simulink model "pmsm_current_loop_discrete"  (R2024b)
settings: Solver=FixedStepDiscrete  StartTime=0.0  StopTime=0.05  FixedStep=Ts  RelTol=1e-3
InitFcn:
  | model_file = get_param(bdroot, 'FileName');
  | model_dir = fileparts(model_file);
  | run(fullfile(model_dir, 'pmsm_current_loop_params.m'));
values from neighbouring files (symbols this model uses):
  flux_wb = 0.0078    [pmsm_current_loop_params.m]
  id_ki = iq_ki * 0.2    (= 666)    [pmsm_current_loop_params.m]
  id_kp = iq_kp * 0.5    (= 1.885)    [pmsm_current_loop_params.m]
  id_ref_after = id_ref_a_default    (= 0)    [pmsm_current_loop_params.m]
  id_ref_before = 0.0    (= 0)    [pmsm_current_loop_params.m]
  id_ref_step_time = 0.001    [pmsm_current_loop_params.m]
  iq_ki = 3330.0    (= 3330)    [pmsm_current_loop_params.m]
  iq_kp = 3.770    (= 3.77)    [pmsm_current_loop_params.m]
  iq_ref_after = iq_ref_a_default    (= 1)    [pmsm_current_loop_params.m]
  iq_ref_before = 0.0    (= 0)    [pmsm_current_loop_params.m]
  iq_ref_step_time = 0.001    [pmsm_current_loop_params.m]
  Ld = 0.0006    [pmsm_current_loop_params.m]
  Lq = 0.0006    [pmsm_current_loop_params.m]
  plant_vd_effect_sign = -1.0    (= -1)    [pmsm_current_loop_params.m]
  plant_vq_effect_sign = -1.0    (= -1)    [pmsm_current_loop_params.m]
  pole_pairs = 4.0    (= 4)    [pmsm_current_loop_params.m]
  pwm_arr = 5311.0    (= 5311)    [pmsm_current_loop_params.m]
  Rs = 0.53    [pmsm_current_loop_params.m]
  sim_mech_speed_rad_s = 50.0    (= 50)    [pmsm_current_loop_params.m]
  svpwm_max_ccr = pwm_arr - 20.0    (= 5291)    [pmsm_current_loop_params.m]
  svpwm_min_ccr = 20.0    (= 20)    [pmsm_current_loop_params.m]
  Ts = 6.25e-5    (= 6.25e-05)    [pmsm_current_loop_params.m]
  use_svpwm_equivalent = 0    [pmsm_current_loop_params.m]
  v_limit = 13.5    [pmsm_current_loop_params.m]
  Vbus = 24.0    (= 24)    [pmsm_current_loop_params.m]
  vd_cmd_sign = -1.0    (= -1)    [pmsm_current_loop_params.m]
  vq_cmd_sign = -1.0    (= -1)    [pmsm_current_loop_params.m]
Description:
  | PMSM discrete current-loop verification model.
  | Parameters are loaded from model/simulink/pmsm_current_loop_params.m.
  | use_svpwm_equivalent=0 bypasses SVPWM and feeds InvPark voltage directly to the plant.
  | use_svpwm_equivalent=1 uses the C-like SVPWM/inverter equivalent before the plant.
  | No observer, PLL, handover, startup, speed loop, or Simscape power bridge is included.
settings Model: Creator=10095  LastModifiedBy=10095
settings DataIOCC: SaveFormat=StructureWithTime

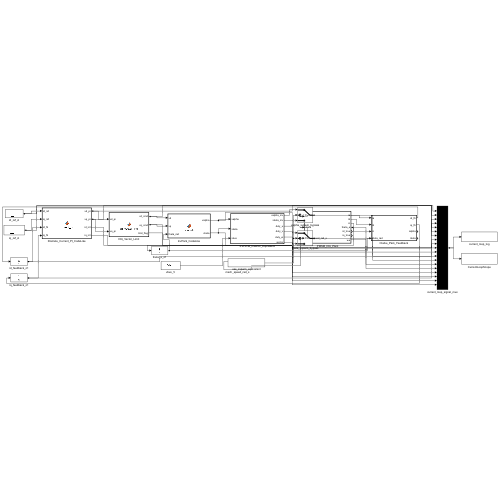
[thumbnail: Simulink's stored preview of the top-level diagram]
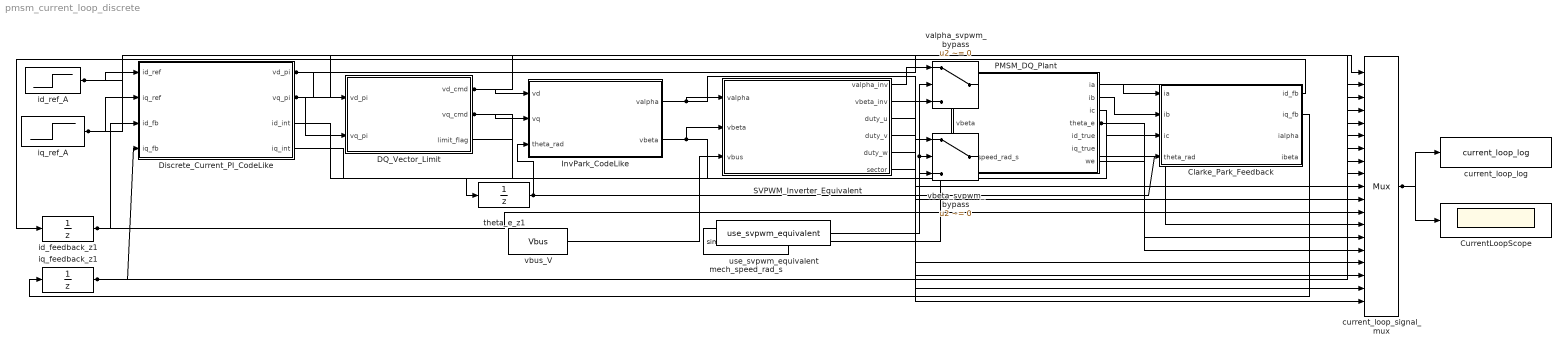
== system pmsm_current_loop_discrete ==
  Clarke_Park_Feedback : MATLAB Function  TreatAsAtomicUnit=on
  CurrentLoopScope : Scope
  DQ_Vector_Limit : MATLAB Function  TreatAsAtomicUnit=on
  Discrete_Current_PI_CodeLike : MATLAB Function  TreatAsAtomicUnit=on
  InvPark_CodeLike : MATLAB Function  TreatAsAtomicUnit=on
  PMSM_DQ_Plant : MATLAB Function  TreatAsAtomicUnit=on
  SVPWM_Inverter_Equivalent : MATLAB Function  TreatAsAtomicUnit=on
  current_loop_log : ToWorkspace  VariableName=current_loop_log  SampleTime=-1
  current_loop_signal_mux : Mux  Inputs=19
  id_feedback_z1 : UnitDelay  SampleTime=Ts  HasFrameUpgradeWarning=on
  id_ref_A : Step  Time=id_ref_step_time  Before=id_ref_before  After=id_ref_after  SampleTime=Ts
  iq_feedback_z1 : UnitDelay  SampleTime=Ts  HasFrameUpgradeWarning=on
  iq_ref_A : Step  Time=iq_ref_step_time  Before=iq_ref_before  After=iq_ref_after  SampleTime=Ts
  mech_speed_rad_s : Constant  Value=sim_mech_speed_rad_s
  theta_e_z1 : UnitDelay  SampleTime=Ts  HasFrameUpgradeWarning=on
  use_svpwm_equivalent : Constant  Value=use_svpwm_equivalent
  valpha_svpwm_bypass : Switch  Criteria=u2 ~= 0  Threshold=0.5  SaturateOnIntegerOverflow=off  InputSameDT=off
  vbeta_svpwm_bypass : Switch  Criteria=u2 ~= 0  Threshold=0.5  SaturateOnIntegerOverflow=off  InputSameDT=off
  vbus_V : Constant  Value=Vbus
  wires:
  id_ref_A/1 -> Discrete_Current_PI_CodeLike/1(id_ref), current_loop_signal_mux/1
  iq_ref_A/1 -> Discrete_Current_PI_CodeLike/2(iq_ref), current_loop_signal_mux/2
  id_feedback_z1/1 -> Discrete_Current_PI_CodeLike/3(id_fb), current_loop_signal_mux/3
  iq_feedback_z1/1 -> Discrete_Current_PI_CodeLike/4(iq_fb), current_loop_signal_mux/4
  Discrete_Current_PI_CodeLike/1(vd_pi) -> DQ_Vector_Limit/1(vd_pi), current_loop_signal_mux/5
  Discrete_Current_PI_CodeLike/2(vq_pi) -> DQ_Vector_Limit/2(vq_pi), current_loop_signal_mux/6
  DQ_Vector_Limit/1(vd_cmd) -> InvPark_CodeLike/1(vd), current_loop_signal_mux/7
  DQ_Vector_Limit/2(vq_cmd) -> InvPark_CodeLike/2(vq), current_loop_signal_mux/8
  theta_e_z1/1 -> InvPark_CodeLike/3(theta_rad), Clarke_Park_Feedback/4(theta_rad)
  InvPark_CodeLike/1(valpha) -> SVPWM_Inverter_Equivalent/1(valpha), valpha_svpwm_bypass/3
  InvPark_CodeLike/2(vbeta) -> SVPWM_Inverter_Equivalent/2(vbeta), vbeta_svpwm_bypass/3
  vbus_V/1 -> SVPWM_Inverter_Equivalent/3(vbus)
  mech_speed_rad_s/1 -> PMSM_DQ_Plant/3(mech_speed_rad_s)
  PMSM_DQ_Plant/1(ia) -> Clarke_Park_Feedback/1(ia)
  PMSM_DQ_Plant/2(ib) -> Clarke_Park_Feedback/2(ib)
  PMSM_DQ_Plant/3(ic) -> Clarke_Park_Feedback/3(ic)
  Clarke_Park_Feedback/1(id_fb) -> id_feedback_z1/1
  Clarke_Park_Feedback/2(iq_fb) -> iq_feedback_z1/1
  PMSM_DQ_Plant/4(theta_e) -> theta_e_z1/1, current_loop_signal_mux/14
  SVPWM_Inverter_Equivalent/1(valpha_inv) -> valpha_svpwm_bypass/1
  use_svpwm_equivalent/1 -> valpha_svpwm_bypass/2, vbeta_svpwm_bypass/2
  SVPWM_Inverter_Equivalent/2(vbeta_inv) -> vbeta_svpwm_bypass/1
  valpha_svpwm_bypass/1 -> PMSM_DQ_Plant/1(valpha), current_loop_signal_mux/12
  vbeta_svpwm_bypass/1 -> PMSM_DQ_Plant/2(vbeta), current_loop_signal_mux/13
  DQ_Vector_Limit/3(limit_flag) -> current_loop_signal_mux/9
  Discrete_Current_PI_CodeLike/3(id_int) -> current_loop_signal_mux/10
  Discrete_Current_PI_CodeLike/4(iq_int) -> current_loop_signal_mux/11
  PMSM_DQ_Plant/7(we) -> current_loop_signal_mux/15
  SVPWM_Inverter_Equivalent/3(duty_u) -> current_loop_signal_mux/16
  SVPWM_Inverter_Equivalent/4(duty_v) -> current_loop_signal_mux/17
  SVPWM_Inverter_Equivalent/5(duty_w) -> current_loop_signal_mux/18
  SVPWM_Inverter_Equivalent/6(sector) -> current_loop_signal_mux/19
  current_loop_signal_mux/1 -> current_loop_log/1, CurrentLoopScope/1

== matlab function pmsm_current_loop_discrete/PMSM_DQ_Plant ==
  data: valpha input; ia output; vbeta input; mech_speed_rad_s input; ib output; ic output; theta_e output; id_true output; iq_true output; we output; pole_pairs parameter; Ts parameter; Rs parameter; Ld parameter; Lq parameter; flux_wb parameter; plant_vd_effect_sign parameter; plant_vq_effect_sign parameter
function [ia, ib, ic, theta_e, id_true, iq_true, we] = pmsm_plant(valpha, vbeta, mech_speed_rad_s, pole_pairs, Ts, Rs, Ld, Lq, flux_wb, plant_vd_effect_sign, plant_vq_effect_sign)
%#codegen
persistent id_state iq_state theta
ia = 0.0; ib = 0.0; ic = 0.0;
theta_e = 0.0; id_true = 0.0; iq_true = 0.0; we = 0.0;
if isempty(id_state)
    id_state = 0.0;
    iq_state = 0.0;
    theta = 0.0;
end
we = pole_pairs * mech_speed_rad_s;
theta_e = theta;
s = sin(theta_e);
c = cos(theta_e);
% C reference: ClarkePark_Park() in foc_clarke_park.c.
vd_cmd = (valpha * c) + (vbeta * s);
vq_cmd = (-valpha * s) + (vbeta * c);
% Plant-side polarity adapter only. The control-side negative signs are
% vd_cmd_sign/vq_cmd_sign in foc_current_loop.c, not hidden here.
vd = plant_vd_effect_sign * vd_cmd;
vq = plant_vq_effect_sign * vq_cmd;
did = (vd - (Rs * id_state) + (we * Lq * iq_state)) / Ld;
diq = (vq - (Rs * iq_state) - (we * Ld * id_state) - (we * flux_wb)) / Lq;
id_state = id_state + (Ts * did);
iq_state = iq_state + (Ts * diq);
theta = theta + (we * Ts);
theta = theta - (floor(theta / 6.283185307179586) * 6.283185307179586);
id_true = id_state;
iq_true = iq_state;
ialpha = (id_state * c) - (iq_state * s);
ibeta = (id_state * s) + (iq_state * c);
ia = ialpha;
ib = (-0.5 * ialpha) + (0.8660254 * ibeta);
ic = (-0.5 * ialpha) - (0.8660254 * ibeta);
end

== matlab function pmsm_current_loop_discrete/Clarke_Park_Feedback ==
  data: ia input; id_fb output; ib input; ic input; theta_rad input; iq_fb output; ialpha output; ibeta output
function [id_fb, iq_fb, ialpha, ibeta] = clarke_park_feedback(ia, ib, ic, theta_rad)
%#codegen
id_fb = 0.0; iq_fb = 0.0; ialpha = 0.0; ibeta = 0.0;
unused_ic = ic;
% C reference: ClarkePark_Clarke() in foc_clarke_park.c.
ialpha = ia;
ibeta = (ia + (2.0 * ib)) * 0.577350269;
s = sin(theta_rad);
c = cos(theta_rad);
% C reference: ClarkePark_Park() in foc_clarke_park.c.
id_fb = (ialpha * c) + (ibeta * s);
iq_fb = (-ialpha * s) + (ibeta * c);
if unused_ic ~= unused_ic
    id_fb = id_fb;
end
end

== matlab function pmsm_current_loop_discrete/DQ_Vector_Limit ==
  data: vd_pi input; vd_cmd output; vq_pi input; vq_cmd output; limit_flag output; dq_v_limit parameter
function [vd_cmd, vq_cmd, limit_flag] = dq_vector_limit(vd_pi, vq_pi, dq_v_limit)
%#codegen
vd_cmd = 0.0; vq_cmd = 0.0; limit_flag = 0.0;
mag_sq = (vd_pi * vd_pi) + (vq_pi * vq_pi);
limit_sq = dq_v_limit * dq_v_limit;
if mag_sq > limit_sq
    scale = dq_v_limit / sqrt(mag_sq);
    vd_cmd = vd_pi * scale;
    vq_cmd = vq_pi * scale;
    limit_flag = 1.0;
else
    vd_cmd = vd_pi;
    vq_cmd = vq_pi;
    limit_flag = 0.0;
end
end

== matlab function pmsm_current_loop_discrete/Discrete_Current_PI_CodeLike ==
  data: id_ref input; vd_pi output; iq_ref input; id_fb input; iq_fb input; vq_pi output; id_int output; iq_int output; id_kp parameter; id_ki parameter; iq_kp parameter; iq_ki parameter; Ts parameter; v_limit parameter; vd_cmd_sign parameter; vq_cmd_sign parameter
function [vd_pi, vq_pi, id_int, iq_int] = current_pi(id_ref, iq_ref, id_fb, iq_fb, id_kp, id_ki, iq_kp, iq_ki, Ts, v_limit, vd_cmd_sign, vq_cmd_sign)
%#codegen
persistent id_integral iq_integral
vd_pi = 0.0; vq_pi = 0.0; id_int = 0.0; iq_int = 0.0;
if isempty(id_integral)
    id_integral = 0.0;
    iq_integral = 0.0;
end
[id_out, id_integral] = pi_run(id_ref, id_fb, id_kp, id_ki, id_integral, Ts, v_limit);
[iq_out, iq_integral] = pi_run(iq_ref, iq_fb, iq_kp, iq_ki, iq_integral, Ts, v_limit);
% C reference: foc_current_loop.c multiplies PI output by FOC_VD_CMD_SIGN.
vd_pi = vd_cmd_sign * id_out;
% C reference: foc_current_loop.c multiplies PI output by FOC_VQ_CMD_SIGN.
vq_pi = vq_cmd_sign * iq_out;
id_int = id_integral;
iq_int = iq_integral;
end

function [out, integral] = pi_run(ref, meas, kp, ki, integral, dt_sec, limit)
err = ref - meas;
p_term = kp * err;
integral_next = integral + (ki * err * dt_sec);
integral_next = clampf(integral_next, -limit, limit);
unsat = p_term + integral_next;
out = clampf(unsat, -limit, limit);
if ((unsat == out) || ((unsat > limit) && (err < 0.0)) || ((unsat < -limit) && (err > 0.0)))
    integral = integral_next;
end
end

function y = clampf(x, mn, mx)
if x > mx
    y = mx;
elseif x < mn
    y = mn;
else
    y = x;
end
end

== matlab function pmsm_current_loop_discrete/InvPark_CodeLike ==
  data: vd input; valpha output; vq input; theta_rad input; vbeta output
function [valpha, vbeta] = invpark(vd, vq, theta_rad)
%#codegen
valpha = 0.0; vbeta = 0.0;
s = sin(theta_rad);
c = cos(theta_rad);
% C reference: ClarkePark_InvPark() in foc_clarke_park.c.
valpha = (vd * c) - (vq * s);
vbeta = (vd * s) + (vq * c);
end

== matlab function pmsm_current_loop_discrete/SVPWM_Inverter_Equivalent ==
  data: valpha input; valpha_inv output; vbeta input; vbus input; vbeta_inv output; duty_u output; duty_v output; duty_w output; sector output; pwm_arr parameter; Vbus parameter; svpwm_min_ccr parameter; svpwm_max_ccr parameter
function [valpha_inv, vbeta_inv, duty_u, duty_v, duty_w, sector] = svpwm_inverter(valpha, vbeta, vbus, pwm_arr, Vbus, svpwm_min_ccr, svpwm_max_ccr)
%#codegen
valpha_inv = 0.0; vbeta_inv = 0.0;
duty_u = 0.5; duty_v = 0.5; duty_w = 0.5; sector = 1.0;
two_pi = 6.283185307179586;
pi_over_3 = 1.047197551196598;
sqrt3 = 1.732050807568877;
pwm_period = pwm_arr;
angle = atan2(vbeta, valpha);
if angle < 0.0
    angle = angle + two_pi;
end
sector = floor(angle * 0.95492965855) + 1.0;
if sector > 6.0
    sector = 6.0;
end
norm_vbus = vbus;
if norm_vbus <= 0.1
    norm_vbus = Vbus;
end
theta_sector = angle - ((sector - 1.0) * pi_over_3);
if theta_sector < 0.0
    theta_sector = 0.0;
elseif theta_sector > pi_over_3
    theta_sector = pi_over_3;
end
vref = sqrt((valpha * valpha) + (vbeta * vbeta));
t1 = pwm_period * sqrt3 * (vref / norm_vbus) * sin(pi_over_3 - theta_sector);
t2 = pwm_period * sqrt3 * (vref / norm_vbus) * sin(theta_sector);
if t1 < 0.0, t1 = 0.0; end
if t2 < 0.0, t2 = 0.0; end
if (t1 + t2) > pwm_period
    scale = pwm_period / (t1 + t2);
    t1 = t1 * scale;
    t2 = t2 * scale;
end
t0 = pwm_period - t1 - t2;
if t0 < 0.0, t0 = 0.0; end
half_t0 = 0.5 * t0;
if sector == 1.0
    ta = t1 + t2 + half_t0; tb = t2 + half_t0;      tc = half_t0;
elseif sector == 2.0
    ta = t1 + half_t0;      tb = t1 + t2 + half_t0; tc = half_t0;
elseif sector == 3.0
    ta = half_t0;           tb = t1 + t2 + half_t0; tc = t2 + half_t0;
elseif sector == 4.0
    ta = half_t0;           tb = t1 + half_t0;      tc = t1 + t2 + half_t0;
elseif sector == 5.0
    ta = t2 + half_t0;      tb = half_t0;           tc = t1 + t2 + half_t0;
else
    ta = t1 + t2 + half_t0; tb = half_t0;           tc = t1 + half_t0;
end
duty_u = clampf(ta / pwm_period, 0.0, 1.0);
duty_v = clampf(tb / pwm_period, 0.0, 1.0);
duty_w = clampf(tc / pwm_period, 0.0, 1.0);
ccr_u = clampf(floor(duty_u * pwm_period), svpwm_min_ccr, svpwm_max_ccr);
ccr_v = clampf(floor(duty_v * pwm_period), svpwm_min_ccr, svpwm_max_ccr);
ccr_w = clampf(floor(duty_w * pwm_period), svpwm_min_ccr, svpwm_max_ccr);
duty_u = ccr_u / pwm_period;
duty_v = ccr_v / pwm_period;
duty_w = ccr_w / pwm_period;
vu = (duty_u - 0.5) * vbus;
vv = (duty_v - 0.5) * vbus;
% C reference: ClarkePark_Clarke() alpha/beta reconstruction convention.
valpha_inv = vu;
vbeta_inv = (vu + (2.0 * vv)) * 0.577350269;
end

function y = clampf(x, mn, mx)
if x > mx
    y = mx;
elseif x < mn
    y = mn;
else
    y = x;
end
end
